simulink model "IFSSIM_Steering"  (R2025b)
settings: Solver=FixedStepDiscrete  StartTime=0  StopTime=inf  FixedStep=1/960  RelTol=1e-3
undefined symbols (not defined in the file or in its folder): IFSSIM_ack, IFSSIM_dmax, IFSSIM_drate, IFSSIM_dtau, IFSSIM_L, IFSSIM_tF, IFSSIM_Ts
settings Model: Creator=raulmoran  LastModifiedBy=raulmoran

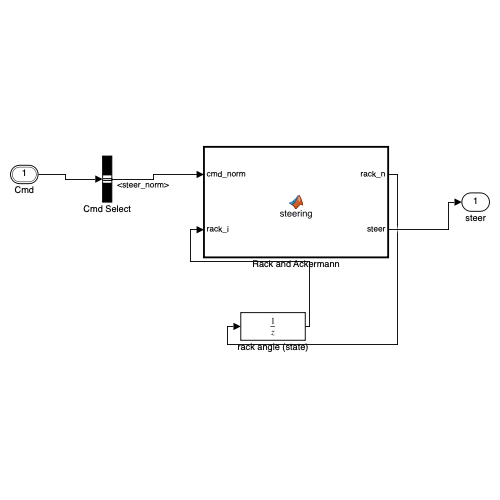
[thumbnail: Simulink's stored preview of the top-level diagram]
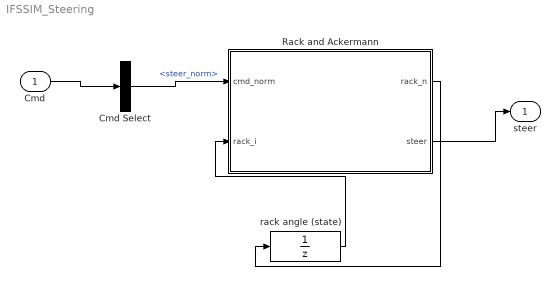
== system IFSSIM_Steering ==
  Cmd : Inport  OutDataTypeStr=Bus: IFSSIM_CmdBus  BusOutputAsStruct=on
  Cmd Select : BusSelector  OutputSignals=steer_norm
  Rack and Ackermann : MATLAB Function  TreatAsAtomicUnit=on
  rack angle (state) : UnitDelay  SampleTime=-1  HasFrameUpgradeWarning=on
  steer : Outport  PortDimensions=4
  wires:
  Cmd/1 -> Cmd Select/1
  Cmd Select/1 -> Rack and Ackermann/1(cmd_norm)  "<steer_norm>"
  rack angle (state)/1 -> Rack and Ackermann/2(rack_i)
  Rack and Ackermann/1(rack_n) -> rack angle (state)/1
  Rack and Ackermann/2(steer) -> steer/1

== matlab function IFSSIM_Steering/Rack and Ackermann ==
  data: cmd_norm input size=1; rack_n output size=1; rack_i input size=1; steer output size=4; IFSSIM_Ts parameter size=1; IFSSIM_dmax parameter size=1; IFSSIM_L parameter size=1; IFSSIM_tF parameter size=1; IFSSIM_ack parameter size=1; IFSSIM_drate parameter size=1; IFSSIM_dtau parameter size=1
function [rack_n, steer] = steering(cmd_norm, rack_i, IFSSIM_Ts, IFSSIM_dmax, IFSSIM_L, IFSSIM_tF, IFSSIM_ack, IFSSIM_drate, IFSSIM_dtau)
%#codegen
% Normalised steering command -> four road-wheel angles.
%
% The rack state is the SINGLE-TRACK (bicycle) angle. Ackermann then splits it
% between the front wheels. The autonomy plans against a kinematic bicycle, so
% this is the definition that keeps the controller's geometry and the plant's
% in agreement.

Ts = IFSSIM_Ts;

% Command -> demanded single-track angle.
cmd = max(-1, min(1, cmd_norm));
target = cmd * IFSSIM_dmax;

% --- actuator ------------------------------------------------------
% First-order lag, then a rate limit. Both default to effectively
% instantaneous — see the note on why an UNMEASURED actuator model is worse
% than none.
alpha = min(Ts / max(IFSSIM_dtau, 1e-9), 1);
lagged = rack_i + alpha * (target - rack_i);

dmax_step = IFSSIM_drate * Ts;
delta = lagged - rack_i;
if delta >  dmax_step, delta =  dmax_step; end
if delta < -dmax_step, delta = -dmax_step; end
rack_n = rack_i + delta;

% --- Ackermann -----------------------------------------------------
% Geometric Ackermann about a common turn centre:
%     R = L / tan(d),  tan(d_inner) = L / (R - t/2),  tan(d_outer) = L / (R + t/2)
% blended toward parallel steer by the Ackermann fraction.
d = rack_i;
if abs(d) < 1e-6
    dl = d; dr = d;                     % straight ahead: no split, and the
                                        % formula below divides by tan(d).
else
    R = IFSSIM_L / tan(d);
    % Positive d steers LEFT in ISO 8855 (y is left, yaw is positive left).
    % The LEFT wheel is then the inner one and takes the larger angle.
    d_in  = atan(IFSSIM_L / (abs(R) - IFSSIM_tF/2));
    d_out = atan(IFSSIM_L / (abs(R) + IFSSIM_tF/2));
    s = sign(d);
    % Blend: 1 = full Ackermann, 0 = both wheels parallel at the rack angle.
    a = IFSSIM_ack;
    d_in_b  = a*d_in  + (1-a)*abs(d);
    d_out_b = a*d_out + (1-a)*abs(d);
    if s > 0
        dl = s*d_in_b;  dr = s*d_out_b;     % turning left: left wheel inner
    else
        dl = s*d_out_b; dr = s*d_in_b;      % turning right: right wheel inner
    end
end

% FL, FR, RL, RR. The rear axle does not steer on this car.
steer = [dl; dr; 0; 0];
end
